simulink model "HDL_pfc_gold_fi_og"  (R2024b)
settings: Solver=FixedStepDiscrete  StartTime=0.0  StopTime=.1  RelTol=1e-3
InitFcn:
  | fidelity_pfc_vals;
  | nbits=(2^12)-2;
  | load('C:\Users\Angel\Desktop\hil\pfc3ph\matlab\sim\sschdl\pfc_desktop\stateSpaceParameters.mat');
values from neighbouring files (symbols this model uses):
  stateSpaceParameters_1 =     [stateSpaceParameters.mat]
undefined symbols (not defined in the file or in its folder): a, b, c, DiscIntNeverNeededParam, Down, Gs, s, t_ss, tsw, Up
libraries: eePwmGenerator x3, dspsrcs4 x3, hdlssclib x2, hdlsllib x1, simulink x1
CloseFcn:
  | clear stateSpaceParameters_1
settings Model: DataTypeOverride=Off  FPTShortcutValueString='{{},{''BaselineRun'',1,1,1,''BaselineRun'','''',{},''M'',''F'',''''}}'  Creator=angro  LastModifiedBy=Angel
settings OptimizationCC: BlockReduction=off  ConditionallyExecuteInputs=off  DefaultParameterBehavior=Inlined  InheritOutputTypeSmallerThanSingle=on  DefaultUnderspecifiedDataType=single
settings DebuggingCC: SignalRangeChecking=warning  AlgebraicLoopMsg=error  ArtificialAlgebraicLoopMsg=error  SingleTaskRateTransMsg=error  UnconnectedInputMsg=warning  UnconnectedOutputMsg=warning  UnconnectedLineMsg=warning
settings HardwareCC: ProdBitPerPointer=32  ProdBitPerSizeT=32  ProdBitPerPtrDiffT=32  ProdLargestAtomicFloat=None  ProdIntDivRoundTo=Undefined  ProdEndianess=Unspecified  ProdWordSize=32  ProdHWDeviceType=ASIC/FPGA->ASIC/FPGA  TargetBitPerPointer=64  TargetBitPerSizeT=64  TargetBitPerPtrDiffT=64  TargetLongLongMode=on  TargetIntDivRoundTo=Zero  TargetEndianess=LittleEndian  TargetWordSize=64  TargetHWDeviceType=Custom Processor->MATLAB Host Computer  ProdEqTarget=off

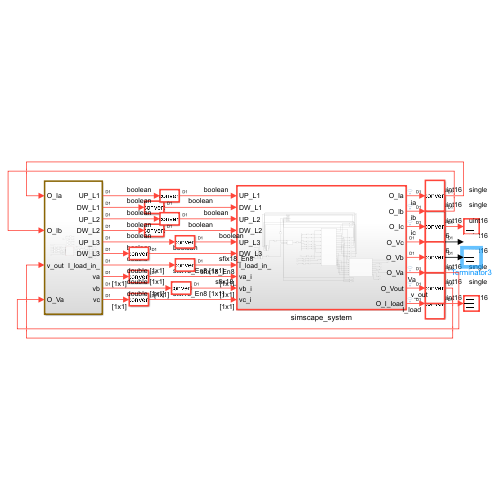
[thumbnail: Simulink's stored preview of the top-level diagram]
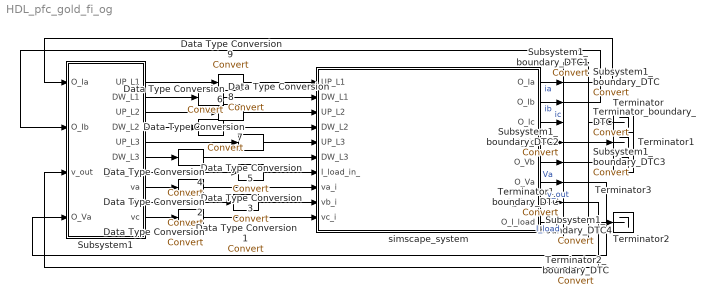
== system HDL_pfc_gold_fi_og ==
  Data Type Conversion{,1..9} (10 alike) : DataTypeConversion  SaturateOnIntegerOverflow=off  RndMeth=Floor
  Subsystem1 : Subsystem
  Subsystem1_boundary_DTC{,1..4} (5 alike) : DataTypeConversion
  Terminator{,1..3} (4 alike) : Terminator
  Terminator1_boundary_DTC : DataTypeConversion
  Terminator2_boundary_DTC : DataTypeConversion
  Terminator_boundary_DTC : DataTypeConversion
  simscape_system : Subsystem
  wires:
  Subsystem1/7(I_load_in_) -> Data Type Conversion3/1
  Subsystem1/1(UP_L1) -> Data Type Conversion9/1
  Subsystem1/2(DW_L1) -> Data Type Conversion8/1
  Subsystem1/3(UP_L2) -> Data Type Conversion7/1
  Subsystem1/4(DW_L2) -> Data Type Conversion6/1
  Subsystem1/5(UP_L3) -> Data Type Conversion5/1
  Subsystem1/6(DW_L3) -> Data Type Conversion4/1
  Subsystem1/8(va) -> Data Type Conversion2/1
  Subsystem1/9(vb) -> Data Type Conversion1/1
  Subsystem1/10(vc) -> Data Type Conversion/1
  Data Type Conversion/1 -> simscape_system/10(vc_i)
  Data Type Conversion1/1 -> simscape_system/9(vb_i)
  Data Type Conversion2/1 -> simscape_system/8(va_i)
  Data Type Conversion3/1 -> simscape_system/7(I_load_in_)
  Data Type Conversion4/1 -> simscape_system/6(DW_L3)
  Data Type Conversion5/1 -> simscape_system/5(UP_L3)
  Data Type Conversion6/1 -> simscape_system/4(DW_L2)
  Data Type Conversion7/1 -> simscape_system/3(UP_L2)
  Data Type Conversion8/1 -> simscape_system/2(DW_L1)
  Data Type Conversion9/1 -> simscape_system/1(UP_L1)
  simscape_system/1(O_Ia) -> Subsystem1_boundary_DTC/1  "ia"
  simscape_system/2(O_Ib) -> Subsystem1_boundary_DTC1/1  "ib"
  simscape_system/3(O_Ic) -> Terminator_boundary_DTC/1  "ic"
  Terminator_boundary_DTC/1 -> Terminator/1
  simscape_system/4(O_Vc) -> Subsystem1_boundary_DTC2/1
  simscape_system/5(O_Vb) -> Subsystem1_boundary_DTC3/1
  simscape_system/6(O_Va) -> Subsystem1_boundary_DTC4/1  "Va"
  simscape_system/7(O_Vout) -> Terminator1_boundary_DTC/1  "v_out"
  Terminator1_boundary_DTC/1 -> Subsystem1/3(v_out)
  simscape_system/8(O_I_load) -> Terminator2_boundary_DTC/1  "I_load"
  Terminator2_boundary_DTC/1 -> Terminator2/1
  Subsystem1_boundary_DTC/1 -> Subsystem1/1(O_Ia)
  Subsystem1_boundary_DTC1/1 -> Subsystem1/2(O_Ib)
  Subsystem1_boundary_DTC4/1 -> Subsystem1/4(O_Va)
  Subsystem1_boundary_DTC2/1 -> Terminator1/1
  Subsystem1_boundary_DTC3/1 -> Terminator3/1

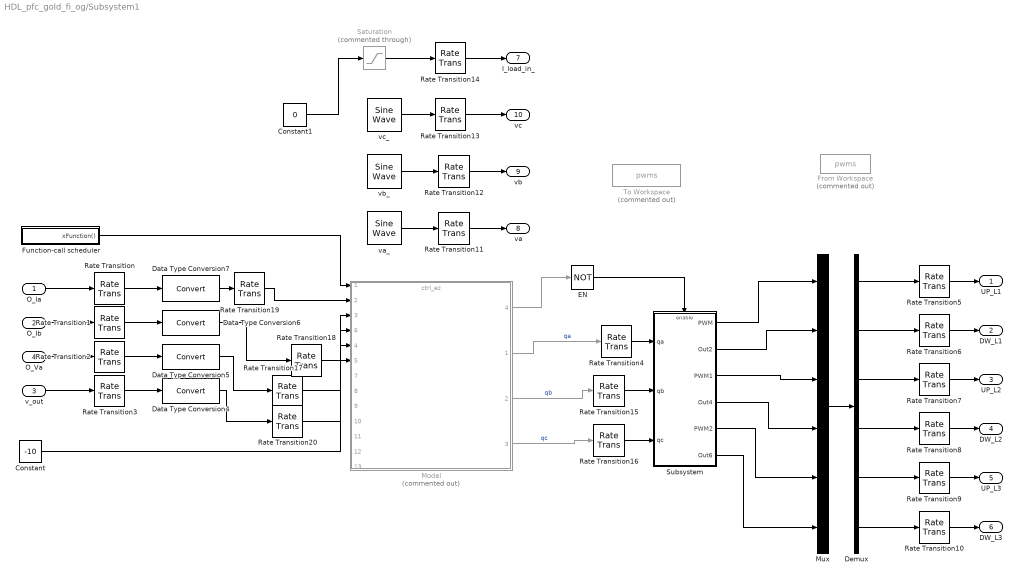
== system HDL_pfc_gold_fi_og/Subsystem1 ==
  O_Ia : Inport
  O_Ib : Inport  Port=2
  v_out : Inport  Port=3
  O_Va : Inport  Port=4
  Constant : Constant  Value=-10  OutDataTypeStr=single  SampleTime=-1
  Constant1 : Constant  Value=0
  Data Type Conversion{4..7} (4 alike) : DataTypeConversion  SaturateOnIntegerOverflow=off  RndMeth=Floor
  Demux : Demux  Outputs=6
  EN : Logic  Operator=NOT  IconShape=distinctive  AllPortsSameDT=off  OutDataTypeStr=boolean
  From Workspace : FromWorkspace  Commented=on  VariableName=pwms
  Function-call scheduler : Test Sequence  TreatAsAtomicUnit=on  SystemSampleTime=tsw
  Model : ModelReference  Commented=on  ModelNameDialog=ctrl_ez.slx  SimulationMode=Normal  ScheduleRates=on  ModelReferenceVersion=1.606
      settings: PortSchema="{\"entries\":[{\"content\":{\"sides\":[{\"content\":{\"connectorIds\":[\"In1\",\"In2\",\"In3\",\"In6\",\"In4\",\"In5\",\"In7\",\"In8\",\"In9\",\"In10\",\"In11\",\"In12\",\"In13\"]},\"type\":\"ConnectorPlacement.EquallySpacedRectSide\",\"uuid\":\"06228333-cac0-4194-8a9e-b8aeb0f2d2c3\"},{\"content\":{\"connectorIds\":[\"Out4\",\"Out1\",\"Out2\",\"Out3\"],\"side\":\"RIGHT\"},\"type\":\"ConnectorPlacement.EquallySpacedRectSide\",\"uuid\":\"40fc62da-d5d1-4d07-aeb6-22788cb15ec8\"},{\"content\":{\"side\":\"TOP\"},\"type\":\"ConnectorPlacement.EquallySpacedRectSide\",\"uuid\":\"88200490-c98c-4a0a-a21b-c8f9cef9ee2d\"}]},\"type\":\"ConnectorPlacement.EquallySpacedConnector\",\"uuid\":\"5f40978a-c38c-41d1-a6a1-03264eebf395\"}],\"packageUris\":[\"http://schema.mathworks.com/mf0/Connector/R2020b\"],\"version\":\"1.0\"}"
  Mux : Mux  Inputs=6
  Rate Transition{,1..3,14} (5 alike) : RateTransition  OutPortSampleTime=t_ss
  Rate Transition{4..13,15..20} (16 alike) : RateTransition
  Saturation : Saturate  Commented=through  UpperLimit=3
  Subsystem : Subsystem
  To Workspace : ToWorkspace  Commented=on  VariableName=pwms  SaveFormat=Timeseries  SampleTime=-1
  va_ : dspsrcs4/Sine Wave  Amplitude=325  Frequency=50  Phase=0  SampleMode=Discrete  OutComplex=Real  CompMethod=Table lookup  TableSize=Speed  SampleTime=tsw  SamplesPerFrame=1  ResetState=Restart at time zero  OutputFrames=off  dataType=double  wordLen=16  udDataType=sfix(16)  fracBitsMode=Best precision  numFracBits=15  OutDataTypeStr=double  LastOutDataTypeStr=double
  vb_ : dspsrcs4/Sine Wave  Amplitude=325  Frequency=50  Phase=(-2*pi/3)  SampleMode=Discrete  OutComplex=Real  CompMethod=Table lookup  TableSize=Speed  SampleTime=tsw  SamplesPerFrame=1  ResetState=Restart at time zero  OutputFrames=off  dataType=double  wordLen=16  udDataType=sfix(16)  fracBitsMode=Best precision  numFracBits=15  OutDataTypeStr=double  LastOutDataTypeStr=double
  vc_ : dspsrcs4/Sine Wave  Amplitude=325  Frequency=50  Phase=(2*pi/3)  SampleMode=Discrete  OutComplex=Real  CompMethod=Table lookup  TableSize=Speed  SampleTime=tsw  SamplesPerFrame=1  ResetState=Restart at time zero  OutputFrames=off  dataType=double  wordLen=16  udDataType=sfix(16)  fracBitsMode=Best precision  numFracBits=15  OutDataTypeStr=double  LastOutDataTypeStr=double
  UP_L1 : Outport
  DW_L1 : Outport  Port=2
  UP_L2 : Outport  Port=3
  DW_L2 : Outport  Port=4
  UP_L3 : Outport  Port=5
  DW_L3 : Outport  Port=6
  I_load_in_ : Outport  Port=7
  va : Outport  Port=8
  vb : Outport  Port=9
  vc : Outport  Port=10
  wires:
  Saturation/1 -> Rate Transition14/1
  Rate Transition10/1 -> DW_L3/1
  Rate Transition14/1 -> I_load_in_/1
  O_Ia/1 -> Rate Transition/1
  O_Va/1 -> Rate Transition2/1
  Rate Transition12/1 -> vb/1
  O_Ib/1 -> Rate Transition1/1
  vb_/1 -> Rate Transition12/1
  Rate Transition6/1 -> DW_L1/1
  v_out/1 -> Rate Transition3/1
  vc_/1 -> Rate Transition13/1
  va_/1 -> Rate Transition11/1
  Demux/5 -> Rate Transition9/1
  Rate Transition11/1 -> va/1
  Demux/4 -> Rate Transition8/1
  Demux/3 -> Rate Transition7/1
  Rate Transition8/1 -> DW_L2/1
  Rate Transition13/1 -> vc/1
  Rate Transition9/1 -> UP_L3/1
  Rate Transition5/1 -> UP_L1/1
  Demux/1 -> Rate Transition5/1
  Demux/2 -> Rate Transition6/1
  Demux/6 -> Rate Transition10/1
  Rate Transition7/1 -> UP_L2/1
  Rate Transition3/1 -> Data Type Conversion4/1
  Rate Transition/1 -> Data Type Conversion7/1
  Rate Transition1/1 -> Data Type Conversion6/1
  Rate Transition2/1 -> Data Type Conversion5/1
  Data Type Conversion7/1 -> Rate Transition19/1
  Data Type Conversion6/1 -> Rate Transition18/1
  Data Type Conversion5/1 -> Rate Transition17/1
  Data Type Conversion4/1 -> Rate Transition20/1
  Constant/1 -> Model/5
  Constant1/1 -> Saturation/1
  Function-call scheduler/1(xFunction()) -> Model/1
  Model/1 -> Rate Transition4/1  "qa"
  Model/2 -> Rate Transition15/1  "qb"
  Model/3 -> Rate Transition16/1  "qc"
  Subsystem/1(PWM) -> Mux/1
  Subsystem/2(Out2) -> Mux/2
  Subsystem/3(PWM1) -> Mux/3
  Subsystem/4(Out4) -> Mux/4
  Subsystem/5(PWM2) -> Mux/5
  Subsystem/6(Out6) -> Mux/6
  Model/4 -> EN/1
  EN/1 -> Subsystem/Enable
  Rate Transition4/1 -> Subsystem/1(qa)
  Rate Transition15/1 -> Subsystem/2(qb)
  Rate Transition16/1 -> Subsystem/3(qc)
  Rate Transition19/1 -> Model/2
  Rate Transition18/1 -> Model/3
  Rate Transition17/1 -> Model/6
  Rate Transition20/1 -> Model/4
  Mux/1 -> Demux/1

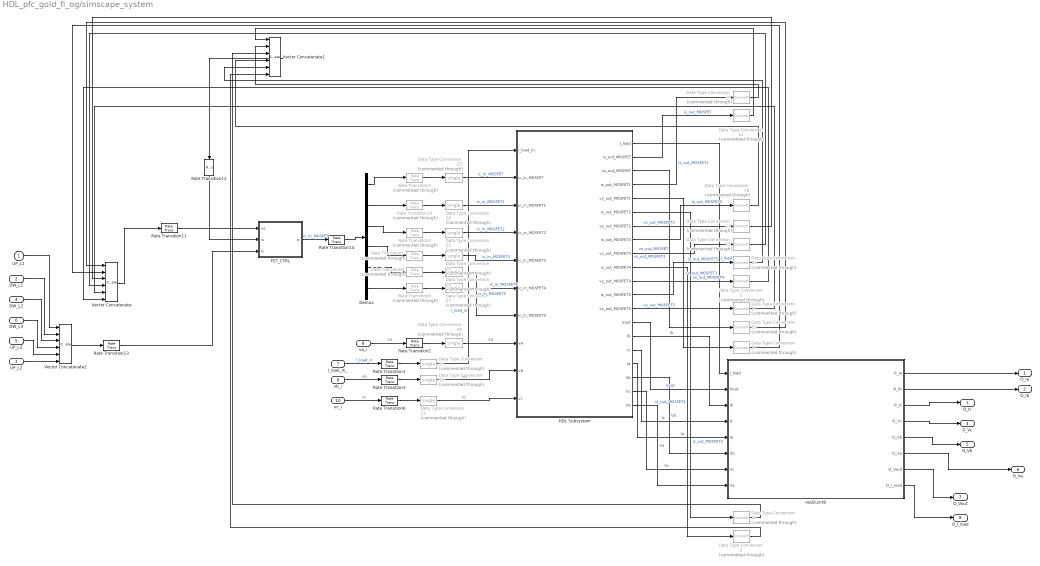
== system HDL_pfc_gold_fi_og/simscape_system ==
  UP_L1 : Inport
  DW_L1 : Inport  Port=2
  UP_L2 : Inport  Port=3
  DW_L2 : Inport  Port=4
  UP_L3 : Inport  Port=5
  DW_L3 : Inport  Port=6
  I_load_in_ : Inport  Port=7  OutDataTypeStr=fixdt(1,18,8)
  va_i : Inport  Port=8  LockScale=on
  vb_i : Inport  Port=9  LockScale=on
  vc_i : Inport  Port=10  LockScale=on
  Data Type Conversion{1..2,10..19} (12 alike) : DataTypeConversion  Commented=through  RndMeth=Nearest  SaturateOnIntegerOverflow=off  LockScale=on
  Data Type Conversion{21..30} (10 alike) : DataTypeConversion  Commented=through  OutDataTypeStr=single  RndMeth=Nearest  SaturateOnIntegerOverflow=off
  Demux : Demux  Outputs=6
  FET_CTRL : Subsystem
  HDL Subsystem : Subsystem
  Rate Transition{1..3,6,11..13} (7 alike) : RateTransition  OutPortSampleTime=t_ss
  Rate Transition{4..5,7..10} (6 alike) : RateTransition  Commented=through  OutPortSampleTime=t_ss
  Rate Transition14 : RateTransition  Integrity=off  OutPortSampleTime=t_ss
  Vector Concatenate : Concatenate  NumInputs=6
  Vector Concatenate1 : Concatenate  NumInputs=6
  Vector Concatenate2 : Concatenate  NumInputs=6
  real2uint8 : Subsystem
  O_Ia : Outport
  O_Ib : Outport  Port=2
  O_Ic : Outport  Port=3
  O_Vc : Outport  Port=4
  O_Vb : Outport  Port=5
  O_Va : Outport  Port=6
  O_Vout : Outport  Port=7
  O_I_load : Outport  Port=8
  wires:
  HDL Subsystem/14(Vout) -> real2uint8/2(Vout)  "Vout"
  HDL Subsystem/13(vs_out_MOSFET5) -> Data Type Conversion11/1  "vs_out_MOSFET5"
  UP_L1/1 -> Vector Concatenate2/1
  HDL Subsystem/16(Ic) -> real2uint8/4(Ic)  "Ic"
  HDL Subsystem/15(Ib) -> real2uint8/3(Ib)  "Ib"
  DW_L1/1 -> Vector Concatenate2/2
  HDL Subsystem/20(Va) -> real2uint8/8(Va)  "Va"
  HDL Subsystem/19(Vc) -> real2uint8/7(Vc)  "Vc"
  DW_L2/1 -> Vector Concatenate2/3
  DW_L3/1 -> Vector Concatenate2/4
  UP_L3/1 -> Vector Concatenate2/5
  HDL Subsystem/18(Vb) -> real2uint8/6(Vb)  "Vb"
  HDL Subsystem/17(Ia) -> real2uint8/5(Ia)  "Ia"
  UP_L2/1 -> Vector Concatenate2/6
  HDL Subsystem/2(is_out_MOSFET) -> Data Type Conversion12/1  "is_out_MOSFET"
  HDL Subsystem/1(I_load) -> real2uint8/1(I_load)  "I_load"
  Vector Concatenate2/1 -> Rate Transition13/1
  FET_CTRL/1(ic) -> Rate Transition14/1  "ic_in_MOSFET"
  I_load_in_/1 -> Rate Transition1/1  "I_load_in"
  Demux/2 -> Rate Transition10/1
  Demux/1 -> Rate Transition7/1
  Rate Transition7/1 -> Data Type Conversion23/1
  va_i/1 -> Rate Transition2/1  "va"
  Demux/4 -> Rate Transition5/1
  Demux/3 -> Rate Transition4/1
  vb_i/1 -> Rate Transition3/1  "vb"
  Demux/6 -> Rate Transition8/1
  Demux/5 -> Rate Transition9/1
  vc_i/1 -> Rate Transition6/1  "vc"
  Rate Transition10/1 -> Data Type Conversion24/1
  Rate Transition4/1 -> Data Type Conversion25/1
  Rate Transition5/1 -> Data Type Conversion26/1
  Data Type Conversion21/1 -> HDL Subsystem/1(I_load_in)  "I_load_in"
  Rate Transition9/1 -> Data Type Conversion28/1
  Rate Transition8/1 -> Data Type Conversion27/1
  Data Type Conversion18/1 -> Vector Concatenate1/4
  Rate Transition2/1 -> Data Type Conversion29/1
  Data Type Conversion24/1 -> HDL Subsystem/3(ic_in_MOSFET1)  "ic_in_MOSFET1"
  Rate Transition1/1 -> Data Type Conversion21/1
  Rate Transition3/1 -> Data Type Conversion30/1
  Data Type Conversion19/1 -> Vector Concatenate1/2
  Rate Transition6/1 -> Data Type Conversion22/1
  Data Type Conversion23/1 -> HDL Subsystem/2(ic_in_MOSFET)  "ic_in_MOSFET"
  Data Type Conversion25/1 -> HDL Subsystem/4(ic_in_MOSFET2)  "ic_in_MOSFET2"
  Data Type Conversion26/1 -> HDL Subsystem/5(ic_in_MOSFET3)  "ic_in_MOSFET3"
  Data Type Conversion28/1 -> HDL Subsystem/7(ic_in_MOSFET5)  "ic_in_MOSFET5"
  Data Type Conversion27/1 -> HDL Subsystem/6(ic_in_MOSFET4)  "ic_in_MOSFET4"
  Data Type Conversion29/1 -> HDL Subsystem/8(va)  "va"
  HDL Subsystem/4(is_out_MOSFET1) -> Data Type Conversion19/1  "is_out_MOSFET1"
  HDL Subsystem/3(vs_out_MOSFET) -> Data Type Conversion10/1  "vs_out_MOSFET"
  Data Type Conversion30/1 -> HDL Subsystem/9(vb)  "vb"
  Data Type Conversion22/1 -> HDL Subsystem/10(vc)  "vc"
  HDL Subsystem/6(is_out_MOSFET2) -> Data Type Conversion16/1  "is_out_MOSFET2"
  HDL Subsystem/5(vs_out_MOSFET1) -> Data Type Conversion17/1  "vs_out_MOSFET1"
  HDL Subsystem/8(is_out_MOSFET3) -> Data Type Conversion18/1  "is_out_MOSFET3"
  HDL Subsystem/7(vs_out_MOSFET2) -> Data Type Conversion14/1  "vs_out_MOSFET2"
  HDL Subsystem/10(is_out_MOSFET4) -> Data Type Conversion2/1  "is_out_MOSFET4"
  HDL Subsystem/9(vs_out_MOSFET3) -> Data Type Conversion15/1  "vs_out_MOSFET3"
  HDL Subsystem/12(is_out_MOSFET5) -> Data Type Conversion13/1  "is_out_MOSFET5"
  HDL Subsystem/11(vs_out_MOSFET4) -> Data Type Conversion1/1  "vs_out_MOSFET4"
  Data Type Conversion12/1 -> Vector Concatenate1/1
  Data Type Conversion14/1 -> Vector Concatenate/3
  Data Type Conversion15/1 -> Vector Concatenate/4
  Data Type Conversion13/1 -> Vector Concatenate1/5
  Data Type Conversion1/1 -> Vector Concatenate/6
  Data Type Conversion11/1 -> Vector Concatenate/5
  Data Type Conversion10/1 -> Vector Concatenate/1
  Data Type Conversion17/1 -> Vector Concatenate/2
  real2uint8/3(O_Ic) -> O_Ic/1
  real2uint8/4(O_Vc) -> O_Vc/1
  real2uint8/5(O_Vb) -> O_Vb/1
  real2uint8/8(O_I_load) -> O_I_load/1
  Data Type Conversion16/1 -> Vector Concatenate1/3
  Data Type Conversion2/1 -> Vector Concatenate1/6
  real2uint8/7(O_Vout) -> O_Vout/1
  Rate Transition13/1 -> FET_CTRL/3(G)
  Vector Concatenate/1 -> Rate Transition11/1
  Vector Concatenate1/1 -> Rate Transition12/1
  Rate Transition14/1 -> Demux/1
  Rate Transition11/1 -> FET_CTRL/1(vs)
  Rate Transition12/1 -> FET_CTRL/2(is)
  real2uint8/1(O_Ia) -> O_Ia/1
  real2uint8/2(O_Ib) -> O_Ib/1
  real2uint8/6(O_Va) -> O_Va/1

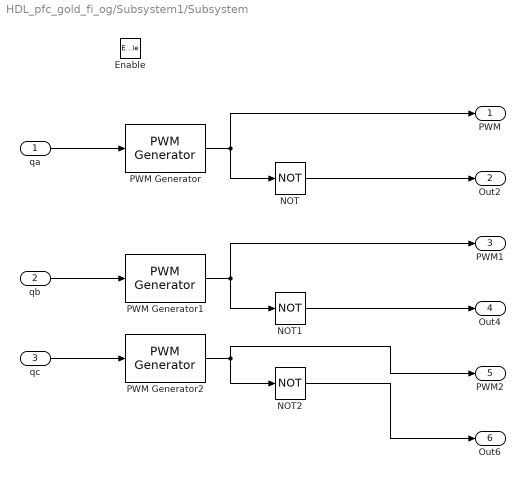
== system HDL_pfc_gold_fi_og/Subsystem1/Subsystem ==
  qa : Inport
  qb : Inport  Port=2
  qc : Inport  Port=3
  Enable : EnablePort
  NOT : Logic  Operator=NOT  IconShape=distinctive  AllPortsSameDT=off  OutDataTypeStr=boolean
  NOT1 : Logic  Operator=NOT  IconShape=distinctive  AllPortsSameDT=off  OutDataTypeStr=boolean
  NOT2 : Logic  Operator=NOT  IconShape=distinctive  AllPortsSameDT=off  OutDataTypeStr=boolean
  PWM Generator : eePwmGenerator/PWM Generator  CarrCount=Up-Down  Tper=tsw  Tdelay=0  Ts=tsw/10
  PWM Generator1 : eePwmGenerator/PWM Generator  CarrCount=Up-Down  Tper=tsw  Tdelay=0  Ts=tsw/10
  PWM Generator2 : eePwmGenerator/PWM Generator  CarrCount=Up-Down  Tper=tsw  Tdelay=0  Ts=tsw/10
  PWM : Outport
  Out2 : Outport  Port=2
  PWM1 : Outport  Port=3
  Out4 : Outport  Port=4
  PWM2 : Outport  Port=5
  Out6 : Outport  Port=6
  wires:
  PWM Generator2/1 -> NOT2/1, PWM2/1
  qc/1 -> PWM Generator2/1
  PWM Generator/1 -> PWM/1, NOT/1
  qa/1 -> PWM Generator/1
  PWM Generator1/1 -> PWM1/1, NOT1/1
  NOT1/1 -> Out4/1
  NOT/1 -> Out2/1
  NOT2/1 -> Out6/1
  qb/1 -> PWM Generator1/1

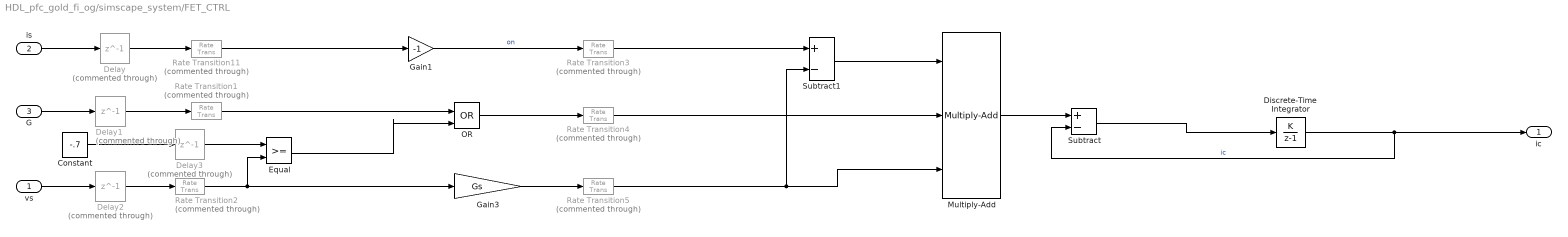
== system HDL_pfc_gold_fi_og/simscape_system/FET_CTRL ==
  vs : Inport  OutDataTypeStr=fixdt(1,18,6)  SampleTime=t_ss
  is : Inport  Port=2  OutDataTypeStr=fixdt(1,18,6)  SampleTime=t_ss
  G : Inport  Port=3  SampleTime=t_ss
  Constant : Constant  Value=-.7  OutDataTypeStr=fixdt(1,18,17)  SampleTime=t_ss
  Delay : Delay  Commented=through  DelayLength=1  InputProcessing=Columns as channels (frame based)  SampleTime=t_ss
  Delay1 : Delay  Commented=through  DelayLength=1  InputProcessing=Columns as channels (frame based)  SampleTime=t_ss
  Delay2 : Delay  Commented=through  DelayLength=1  InputProcessing=Columns as channels (frame based)  SampleTime=t_ss
  Delay3 : Delay  Commented=through  DelayLength=1  InitialCondition=-.7  InputProcessing=Columns as channels (frame based)  SampleTime=t_ss
  Discrete-Time Integrator : DiscreteIntegrator  IntegratorMethod=Accumulation: Forward Euler  gainval=1/s  SampleTime=t_ss  OutDataTypeStr=fixdt(1,18,8)  SaturateOnIntegerOverflow=on  LimitOutput=on  UpperSaturationLimit=100  LowerSaturationLimit=-100  ICPrevOutput=DiscIntNeverNeededParam  ICPrevScaledInput=DiscIntNeverNeededParam
  Equal : RelationalOperator  OutDataTypeStr=boolean  RndMeth=Simplest  InputSameDT=off
  Gain1 : Gain  Gain=-1  OutDataTypeStr=fixdt(1,18,12)
  Gain3 : Gain  Gain=Gs  OutDataTypeStr=fixdt(1,18,12)
  Multiply-Add : hdlsllib/HDL Operations/Multiply-Add  Function=c+(a.*b)  datatype=fixdt(1,18,12)  DoSatur=on  FMA=off
  OR : Logic  Operator=OR  IconShape=distinctive  AllPortsSameDT=off  OutDataTypeStr=boolean
  Rate Transition{1..5,11} (6 alike) : RateTransition  Commented=through  OutPortSampleTime=t_ss
  Subtract : Sum  Inputs=+-  OutDataTypeStr=fixdt(1,18,12)
  Subtract1 : Sum  Inputs=+-  OutDataTypeStr=fixdt(1,18,11)
  ic : Outport  SampleTime=t_ss
  wires:
  OR/1 -> Rate Transition4/1
  Subtract1/1 -> Multiply-Add/1
  Gain3/1 -> Rate Transition5/1
  Constant/1 -> Delay3/1
  Equal/1 -> OR/2
  Subtract/1 -> Discrete-Time Integrator/1
  Discrete-Time Integrator/1 -> ic/1, Subtract/2  "ic"
  Gain1/1 -> Rate Transition3/1  "on"
  Multiply-Add/1 -> Subtract/1
  is/1 -> Delay/1
  G/1 -> Delay1/1
  vs/1 -> Delay2/1
  Delay/1 -> Rate Transition11/1
  Delay1/1 -> Rate Transition1/1
  Delay2/1 -> Rate Transition2/1
  Rate Transition11/1 -> Gain1/1
  Rate Transition1/1 -> OR/1
  Rate Transition2/1 -> Gain3/1, Equal/2
  Delay3/1 -> Equal/1
  Rate Transition3/1 -> Subtract1/1
  Rate Transition4/1 -> Multiply-Add/2
  Rate Transition5/1 -> Multiply-Add/3, Subtract1/2

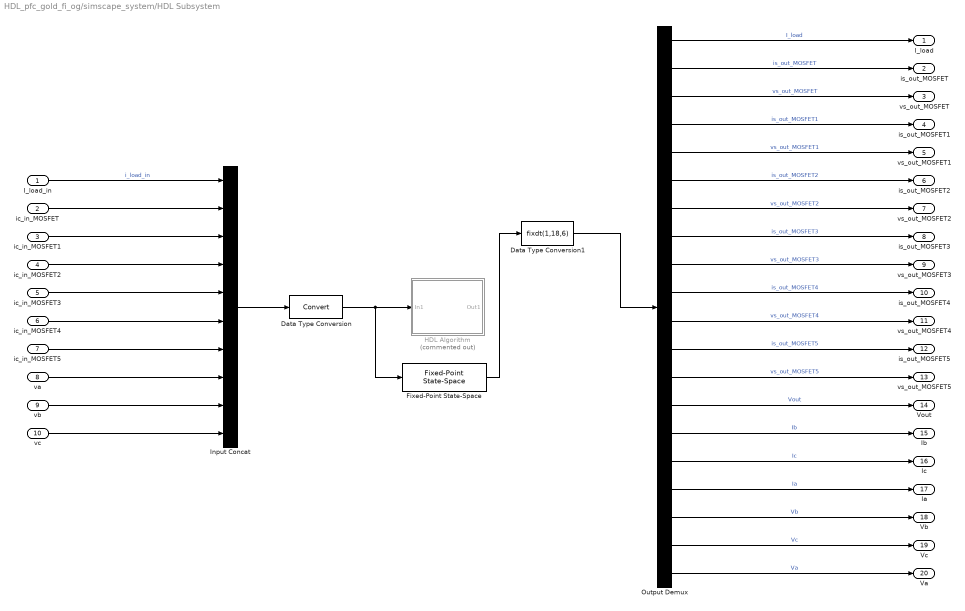
== system HDL_pfc_gold_fi_og/simscape_system/HDL Subsystem ==
  I_load_in : Inport  OutDataTypeStr=fixdt(1,18,8)
  ic_in_MOSFET : Inport  Port=2  OutDataTypeStr=fixdt(1,18,8)
  ic_in_MOSFET1 : Inport  Port=3  OutDataTypeStr=fixdt(1,18,8)
  ic_in_MOSFET2 : Inport  Port=4  OutDataTypeStr=fixdt(1,18,8)
  ic_in_MOSFET3 : Inport  Port=5  OutDataTypeStr=fixdt(1,18,8)
  ic_in_MOSFET4 : Inport  Port=6  OutDataTypeStr=fixdt(1,18,8)
  ic_in_MOSFET5 : Inport  Port=7  OutDataTypeStr=fixdt(1,18,8)
  va : Inport  Port=8  OutDataTypeStr=fixdt(1,18,8)
  vb : Inport  Port=9  OutDataTypeStr=fixdt(1,18,8)
  vc : Inport  Port=10  OutDataTypeStr=fixdt(1,18,8)
  Data Type Conversion : DataTypeConversion  SaturateOnIntegerOverflow=off  RndMeth=Floor
  Data Type Conversion1 : DataTypeConversion  OutDataTypeStr=fixdt(1,18,6)  SaturateOnIntegerOverflow=off  RndMeth=Floor
  Fixed-Point State-Space : simulink/Additional Math & Discrete/Additional Discrete/Fixed-Point State-Space  A=fi(stateSpaceParameters_1.Ad,1,25,24)  B=fi(stateSpaceParameters_1.Bd,1,25,31)  C=fi(stateSpaceParameters_1.Cd,1,25,20)  D=fi(stateSpaceParameters_1.Dd,1,25,19)  InitialCondition=fi(stateSpaceParameters_1.X0,1,25,14)  InternalDataType=fixdt(1,25,13)  StateEqScaling=2^0  OutputEqScaling=2^0  DoSatur=off
  HDL Algorithm : Subsystem  Commented=on
  Input Concat : Concatenate  NumInputs=10
  Output Demux : Demux  Outputs=20
  I_load : Outport
  is_out_MOSFET : Outport  Port=2
  vs_out_MOSFET : Outport  Port=3
  is_out_MOSFET1 : Outport  Port=4
  vs_out_MOSFET1 : Outport  Port=5
  is_out_MOSFET2 : Outport  Port=6
  vs_out_MOSFET2 : Outport  Port=7
  is_out_MOSFET3 : Outport  Port=8
  vs_out_MOSFET3 : Outport  Port=9
  is_out_MOSFET4 : Outport  Port=10
  vs_out_MOSFET4 : Outport  Port=11
  is_out_MOSFET5 : Outport  Port=12
  vs_out_MOSFET5 : Outport  Port=13
  Vout : Outport  Port=14
  Ib : Outport  Port=15
  Ic : Outport  Port=16
  Ia : Outport  Port=17
  Vb : Outport  Port=18
  Vc : Outport  Port=19
  Va : Outport  Port=20
  wires:
  Output Demux/7 -> vs_out_MOSFET2/1  "vs_out_MOSFET2"
  Output Demux/2 -> is_out_MOSFET/1  "is_out_MOSFET"
  Output Demux/3 -> vs_out_MOSFET/1  "vs_out_MOSFET"
  Output Demux/4 -> is_out_MOSFET1/1  "is_out_MOSFET1"
  ic_in_MOSFET/1 -> Input Concat/2
  Input Concat/1 -> Data Type Conversion/1
  Output Demux/17 -> Ia/1  "Ia"
  Output Demux/1 -> I_load/1  "I_load"
  vc/1 -> Input Concat/10
  Output Demux/6 -> is_out_MOSFET2/1  "is_out_MOSFET2"
  Output Demux/8 -> is_out_MOSFET3/1  "is_out_MOSFET3"
  Output Demux/15 -> Ib/1  "Ib"
  Output Demux/13 -> vs_out_MOSFET5/1  "vs_out_MOSFET5"
  Output Demux/5 -> vs_out_MOSFET1/1  "vs_out_MOSFET1"
  Output Demux/12 -> is_out_MOSFET5/1  "is_out_MOSFET5"
  Output Demux/10 -> is_out_MOSFET4/1  "is_out_MOSFET4"
  Output Demux/9 -> vs_out_MOSFET3/1  "vs_out_MOSFET3"
  Output Demux/11 -> vs_out_MOSFET4/1  "vs_out_MOSFET4"
  Output Demux/14 -> Vout/1  "Vout"
  Output Demux/16 -> Ic/1  "Ic"
  Output Demux/19 -> Vc/1  "Vc"
  Output Demux/18 -> Vb/1  "Vb"
  Output Demux/20 -> Va/1  "Va"
  vb/1 -> Input Concat/9
  ic_in_MOSFET1/1 -> Input Concat/3
  I_load_in/1 -> Input Concat/1  "i_load_in"
  ic_in_MOSFET3/1 -> Input Concat/5
  ic_in_MOSFET2/1 -> Input Concat/4
  ic_in_MOSFET5/1 -> Input Concat/7
  va/1 -> Input Concat/8
  ic_in_MOSFET4/1 -> Input Concat/6
  Data Type Conversion1/1 -> Output Demux/1
  Data Type Conversion/1 -> Fixed-Point State-Space/1, HDL Algorithm/1(In1)
  Fixed-Point State-Space/1 -> Data Type Conversion1/1

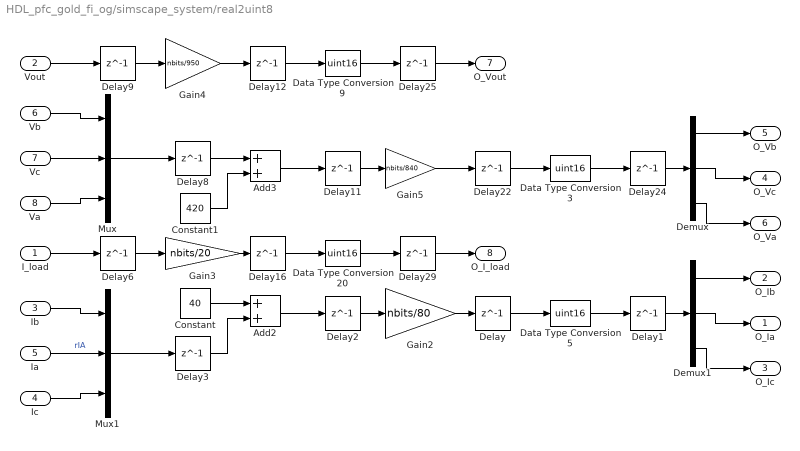
== system HDL_pfc_gold_fi_og/simscape_system/real2uint8 ==
  I_load : Inport
  Vout : Inport  Port=2
  Ib : Inport  Port=3
  Ic : Inport  Port=4
  Ia : Inport  Port=5
  Vb : Inport  Port=6
  Vc : Inport  Port=7
  Va : Inport  Port=8
  Add2 : Sum  OutDataTypeStr=Inherit: Same as first input
  Add3 : Sum
  Constant : Constant  Value=40  OutDataTypeStr=fixdt(1,18,6)  SampleTime=-1
  Constant1 : Constant  Value=420  OutDataTypeStr=fixdt(1,18,6)  SampleTime=-1
  Data Type Conversion{3,5,9,20} (4 alike) : DataTypeConversion  OutDataTypeStr=uint16  RndMeth=Nearest  SaturateOnIntegerOverflow=off  LockScale=on
  Delay{,1..3,6,8..9,11..12,16,22,24..25,29} (14 alike) : Delay  DelayLength=1
  Demux : Demux  Outputs=3
  Demux1 : Demux  Outputs=3
  Gain2 : Gain  Gain=nbits/80  OutDataTypeStr=Inherit: Same as input
  Gain3 : Gain  Gain=nbits/20  OutDataTypeStr=Inherit: Same as input
  Gain4 : Gain  Gain=nbits/950  OutDataTypeStr=Inherit: Same as input
  Gain5 : Gain  Gain=nbits/840  OutDataTypeStr=Inherit: Same as input
  Mux : Mux  Inputs=3
  Mux1 : Mux  Inputs=3
  O_Ia : Outport
  O_Ib : Outport  Port=2
  O_Ic : Outport  Port=3
  O_Vc : Outport  Port=4
  O_Vb : Outport  Port=5
  O_Va : Outport  Port=6
  O_Vout : Outport  Port=7
  O_I_load : Outport  Port=8
  wires:
  Add2/1 -> Delay2/1
  Va/1 -> Mux/3
  Ic/1 -> Mux1/3
  Data Type Conversion9/1 -> Delay25/1
  Vout/1 -> Delay9/1
  Vb/1 -> Mux/1
  Ia/1 -> Mux1/2  "rIA"
  Gain5/1 -> Delay22/1
  Vc/1 -> Mux/2
  Ib/1 -> Mux1/1
  Delay11/1 -> Gain5/1
  I_load/1 -> Delay6/1
  Demux/1 -> O_Vb/1
  Delay29/1 -> O_I_load/1
  Delay9/1 -> Gain4/1
  Mux/1 -> Delay8/1
  Delay6/1 -> Gain3/1
  Mux1/1 -> Delay3/1
  Gain4/1 -> Delay12/1
  Delay2/1 -> Gain2/1
  Delay8/1 -> Add3/1
  Constant1/1 -> Add3/2
  Gain3/1 -> Delay16/1
  Constant/1 -> Add2/1
  Delay3/1 -> Add2/2
  Delay12/1 -> Data Type Conversion9/1
  Add3/1 -> Delay11/1
  Delay16/1 -> Data Type Conversion20/1
  Data Type Conversion20/1 -> Delay29/1
  Delay25/1 -> O_Vout/1
  Gain2/1 -> Delay/1
  Delay22/1 -> Data Type Conversion3/1
  Delay24/1 -> Demux/1
  Delay/1 -> Data Type Conversion5/1
  Data Type Conversion3/1 -> Delay24/1
  Data Type Conversion5/1 -> Delay1/1
  Delay1/1 -> Demux1/1
  Demux/2 -> O_Vc/1
  Demux/3 -> O_Va/1
  Demux1/3 -> O_Ic/1
  Demux1/1 -> O_Ib/1
  Demux1/2 -> O_Ia/1

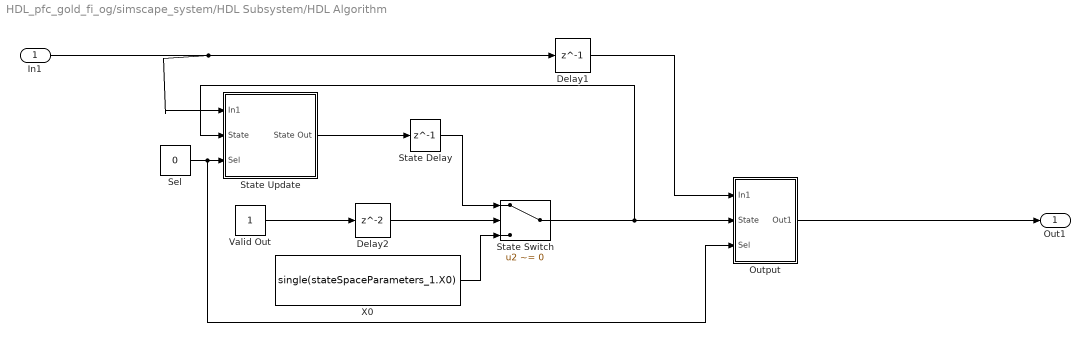
== system HDL_pfc_gold_fi_og/simscape_system/HDL Subsystem/HDL Algorithm ==
  In1 : Inport
  Delay1 : Delay  DelayLength=1
  Delay2 : Delay
  Output : Subsystem
  Sel : Constant  Value=0  OutDataTypeStr=uint32  SampleTime=-1
  State Delay : Delay  DelayLength=1  InitialCondition=single(stateSpaceParameters_1.X0)
  State Switch : Switch  Criteria=u2 ~= 0  SaturateOnIntegerOverflow=off  InputSameDT=off
  State Update : Subsystem
  Valid Out : Constant  OutDataTypeStr=boolean  SampleTime=4.395604395604395e-07
  X0 : Constant  Value=single(stateSpaceParameters_1.X0)  SampleTime=4.395604395604395e-07
  Out1 : Outport  VectorParamsAs1DForOutWhenUnconnected=off
  wires:
  Delay1/1 -> Output/1(In1)
  Sel/1 -> Output/3(Sel), State Update/3(Sel)
  State Update/1(State Out) -> State Delay/1
  Valid Out/1 -> Delay2/1
  State Delay/1 -> State Switch/1
  Delay2/1 -> State Switch/2
  X0/1 -> State Switch/3
  Output/1(Out1) -> Out1/1
  State Switch/1 -> Output/2(State), State Update/2(State)
  In1/1 -> Delay1/1, State Update/1(In1)

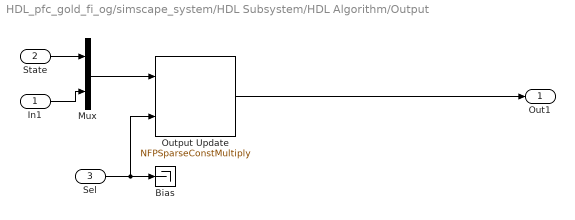
== system HDL_pfc_gold_fi_og/simscape_system/HDL Subsystem/HDL Algorithm/Output ==
  In1 : Inport
  State : Inport  Port=2
  Sel : Inport  Port=3  LockScale=on
  Bias : Terminator
  Mux : Mux  Inputs=2
  Output Update : hdlssclib/NFPSparseConstMultiply  MatrixSource=Dialog  constMatrix=single([stateSpaceParameters_1.Cd stateSpaceParameters_1.Dd])  MatrixType=single  MatrixSize=[1 1]  ColumnIndices=[1]  RowIndices=[1]  PropDataType=single  defWL=48
  Out1 : Outport  VectorParamsAs1DForOutWhenUnconnected=off
  wires:
  State/1 -> Mux/1
  Mux/1 -> Output Update/1
  In1/1 -> Mux/2
  Sel/1 -> Bias/1, Output Update/2
  Output Update/1 -> Out1/1

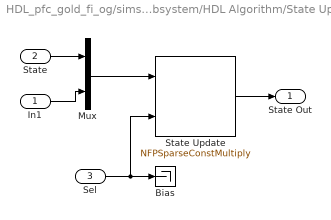
== system HDL_pfc_gold_fi_og/simscape_system/HDL Subsystem/HDL Algorithm/State Update ==
  In1 : Inport
  State : Inport  Port=2
  Sel : Inport  Port=3  LockScale=on
  Bias : Terminator
  Mux : Mux  Inputs=2
  State Update : hdlssclib/NFPSparseConstMultiply  MatrixSource=Dialog  constMatrix=single([stateSpaceParameters_1.Ad stateSpaceParameters_1.Bd])  MatrixType=single  MatrixSize=[1 1]  ColumnIndices=[1]  RowIndices=[1]  PropDataType=single  defWL=43
  State Out : Outport  VectorParamsAs1DForOutWhenUnconnected=off
  wires:
  State/1 -> Mux/1
  In1/1 -> Mux/2
  Mux/1 -> State Update/1
  Sel/1 -> Bias/1, State Update/2
  State Update/1 -> State Out/1

== stateflow chart HDL_pfc_gold_fi_og/Subsystem1/Function-call scheduler ==
  state Run
    send(xFunction);
  (default) -> Run
  events: xFunction output FUNCTION_CALL_EVENT
